simulink model "cic_test2"  (Simulink 6.6)
settings: Solver=FixedStepDiscrete  SolverMode=SingleTasking  StartTime=0.0  StopTime=100  RelTol=1e-3
libraries: dspsigops x7, dspsrcs4 x1
settings Model: Creator=svenhoffmann  LastModifiedBy=svenhoffmann  ExtModeAutoUpdateStatusClock=off
settings OptimizationCC: InlineInvariantSignals=on
settings DebuggingCC: SignalResolutionControl=TryResolveAllWithWarning  MultiTaskDSMMsg=warning  MultiTaskCondExecSysMsg=none  StrictBusMsg=None
settings RTWCC: IncludeERTFirstTime=on

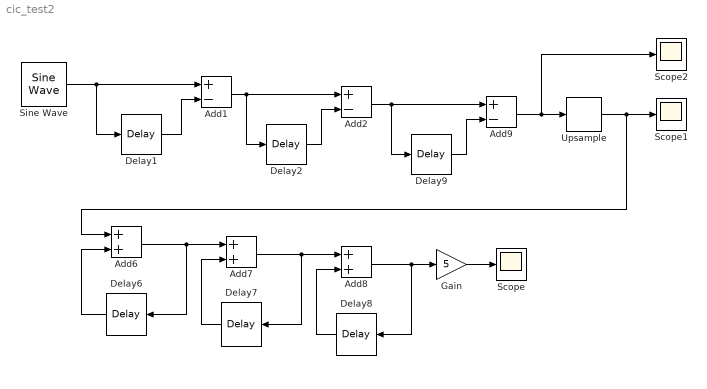
== system cic_test2 ==
  Add1 : Sum  Inputs=+-  OutDataTypeMode=int32  OutScaling=2^-10
  Add2 : Sum  Inputs=+-  OutScaling=2^-10
  Add6 : Sum  OutScaling=2^-10
  Add7 : Sum  OutScaling=2^-10
  Add8 : Sum  OutScaling=2^-10
  Add9 : Sum  Inputs=+-  OutScaling=2^-10
  Delay1 : dspsigops/Delay  dly_unit=Samples  delay=1  ic_detail=off  dif_ic_for_ch=off  dif_ic_for_dly=off  ic=0  reset_popup=None
  Delay2 : dspsigops/Delay  dly_unit=Samples  delay=1  ic_detail=off  dif_ic_for_ch=off  dif_ic_for_dly=off  ic=0  reset_popup=None
  Delay6 : dspsigops/Delay  Orientation=left  dly_unit=Samples  delay=1  ic_detail=off  dif_ic_for_ch=off  dif_ic_for_dly=off  ic=0  reset_popup=None
  Delay7 : dspsigops/Delay  Orientation=left  dly_unit=Samples  delay=1  ic_detail=off  dif_ic_for_ch=off  dif_ic_for_dly=off  ic=0  reset_popup=None
  Delay8 : dspsigops/Delay  Orientation=left  dly_unit=Samples  delay=1  ic_detail=off  dif_ic_for_ch=off  dif_ic_for_dly=off  ic=0  reset_popup=None
  Delay9 : dspsigops/Delay  dly_unit=Samples  delay=1  ic_detail=off  dif_ic_for_ch=off  dif_ic_for_dly=off  ic=0  reset_popup=None
  Gain : Gain  Gain=5
  Scope : Scope
      settings: YMin=-1.25e+08  YMax=1.25e+08
  Scope1 : Scope
      settings: YMin=-12500  YMax=12500
  Scope2 : Scope
      settings: YMin=-2500  YMax=2500  SaveName=ScopeData2
  Sine Wave : dspsrcs4/Sine Wave  Amplitude=2^15  Frequency=5  Phase=0  SampleMode=Discrete  OutComplex=Real  CompMethod=Table lookup  TableSize=Speed  SampleTime=1/100  SamplesPerFrame=1  dataType=Fixed-point  wordLen=16  udDataType=sfix(32)  fracBitsMode=User-defined  numFracBits=0  ResetState=Restart at time zero
  Upsample : dspsigops/Upsample  N=25  phase=0  ic=0  mode=Maintain input frame size
  wires:
  Upsample/1 -> Scope1/1, Add6/1
  Add8/1 -> Delay8/1, Gain/1
  Sine Wave/1 -> Add1/1, Delay1/1
  Delay6/1 -> Add6/2
  Add6/1 -> Delay6/1, Add7/1
  Delay7/1 -> Add7/2
  Add7/1 -> Delay7/1, Add8/1
  Delay8/1 -> Add8/2
  Delay1/1 -> Add1/2
  Delay2/1 -> Add2/2
  Add1/1 -> Delay2/1, Add2/1
  Delay9/1 -> Add9/2
  Add2/1 -> Add9/1, Delay9/1
  Add9/1 -> Upsample/1, Scope2/1
  Gain/1 -> Scope/1
